simulink model "DatePersonalizate"  (R2023b)
settings: Solver=ode3  StartTime=0.0  StopTime=1000  FixedStep=0.1  RelTol=1e-3
values from neighbouring files (symbols this model uses):
  C = 7.4    [date_personalizate.m]
  k = 0.036    [date_personalizate.m]    (also in grafice.m = 0.035)
  k1 = 0.624    [date_personalizate.m]    (also in grafice.m)
  k11 = k2^2+4*(k-k3)*k1    (= 0.0915786)    [date_personalizate.m]
  k12 = 8*(k-k3)    (= 0.2928)    [date_personalizate.m]
  k13 = 2*(k-k3)    (= 0.0732)    [date_personalizate.m]
  k2 = -0.015    [date_personalizate.m]    (also in grafice.m)
  k3 = -0.0006    [date_personalizate.m]    (also in grafice.m)
  keta = 8e-5    (= 8e-05)    [date_personalizate.m]
  S = 332.5    [date_personalizate.m]
libraries: slpidlib x14, instrumentlib x2, simulink x1
(part 1 of 2)
settings Model: Creator=40787  LastModifiedBy=40787
settings GRTTargetCC: RTWCAPISignals=on  RTWCAPIParams=on

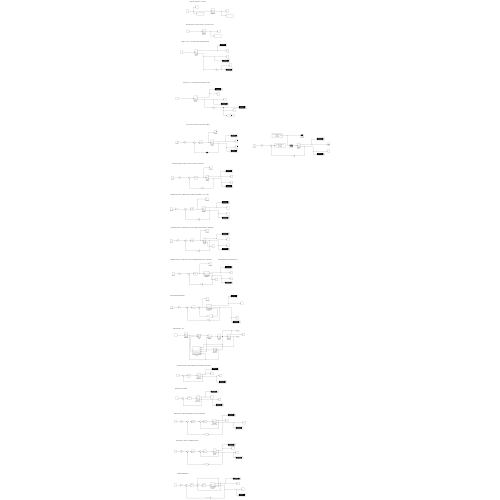
[thumbnail: Simulink's stored preview of the top-level diagram]
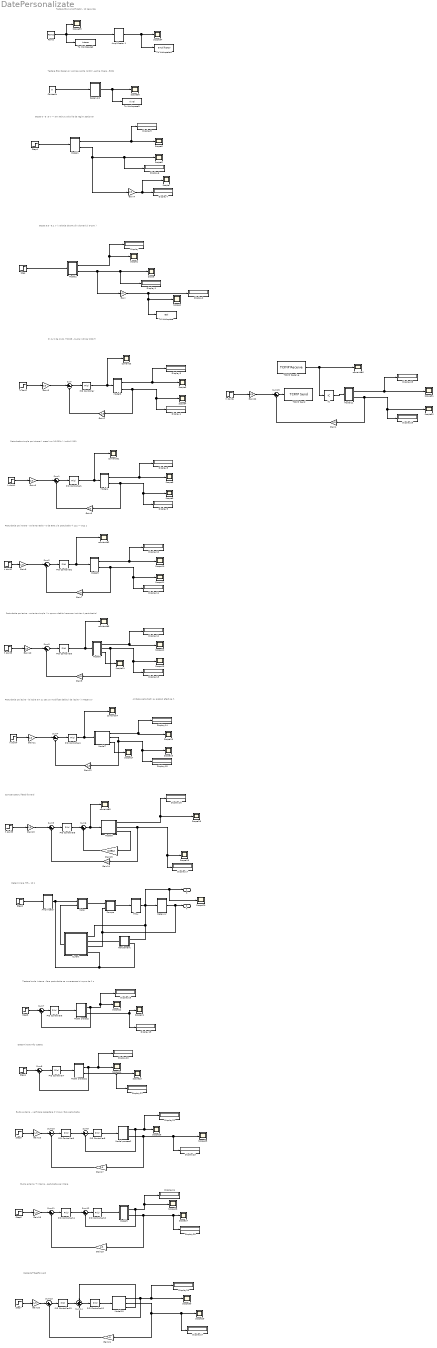
== system DatePersonalizate ==
  note: Testare Bloc Rezervor: pompa oprita (qi=0) - golire libera - 500s
  note: Testare Bloc Amplificator - 10 secunde
  note: trepta 0 - 5 .6 V -> am retinut valorile de regim stationar
  note: trepta 5.6 - 6.1 V ( variatie de 5% din domeniul 0-10V )
  note: PI cu tr de 112s, T0=28 - bucla inchisa (202/7)
  note: Perturbatie simpla pe intrare-> cresc k cu 10-20%-> inchid V101
  note: Perturbatie pe intrare - varianta reala - tr de 800 s la pertubatie + 112 -> 912 s
  note: Perturbatie pe iesire - varianta simpla ( in qe am debitul care era inainte + perturbatia)
  note: Perturbatie pe iesire - la iesire am cu cat s a modificat debitul de iesire - in Rezervor
  note: Compensatorul feed forward
  note: Determinare Hf1 - 10 s
  note: Testare bucla interna - fara perturbatie sa urmareasca tr impus de 1 s
  note: Determinare Hf2 -2500s
  note: Bucla externa - verificare respectare tr impus, fara perturbatie
  note: Bucla externa + interna - pertubatie pe intrare
  note: Cascada+feedforward
  note: Ambele perturbatii au acelasi efect pe h
  "Amplificator " : Subsystem
  Amplificator 1 : Subsystem
  Constant : Constant  Value=0
  Curent : Subsystem
  Display{,1..29} (30 alike) : Display
  Filtru : Subsystem
  Gain{,1..14,16..22} (22 alike) : Gain  Gain=1/3
  Gain15 : Gain  Gain=0.0912
  IC : InitialCondition  Value=5.6
  Model process : Subsystem
  Model process1 : Subsystem
  Model process2 : Subsystem
  Model1 : Subsystem
  Model10 : Subsystem
  Model11 : Subsystem
  Model2 : Subsystem
  Model3 : Subsystem
  Model4 : Subsystem
  Model5 : Subsystem
  Model6 : Subsystem
  Model7 : Subsystem
  Model8 : Subsystem
  Model9 : Subsystem
  Motor : Subsystem
  PID Controller{,1..5} (6 alike) : slpidlib/PID Controller  Controller=PI  Form=Parallel  TimeDomain=Continuous-time  UseExternalTs=off  SampleTime=-1  IntegratorMethod=Forward Euler  FilterMethod=Forward Euler  ControllerParametersSource=internal  P=2.96  I=2.96/202  UseKiTs=off  D=0  N=100  UseFilter=on  TunerSelectOption=Frequency Response Based  InitialConditionSource=internal  InitialConditionForIntegrator=5.6  InitialConditionForFilter=0  DifferentiatorICPrevScaledInput=0  ExternalReset=none  TrackingMode=off  Kt=1  LimitOutput=off  SatLimitsSource=internal  UpperSaturationLimit=inf  LowerSaturationLimit=-inf  LinearizeAsGain=on  AntiWindupMode=none  Kb=1  LimitIntegrator=off  UpperIntegratorSaturationLimit=inf  LowerIntegratorSaturationLimit=-inf  POutMin=[]  POutMax=[]  IOutMin=[]  IOutMax=[]  DOutMin=[]  DOutMax=[]  NOutMin=[]  NOutMax=[]  SumOutMin=[]  SumOutMax=[]  SaturationOutMin=[]  SaturationOutMax=[]  PParamMin=[]  PParamMax=[]  IParamMin=[]  IParamMax=[]  DParamMin=[]  DParamMax=[]  NParamMin=[]  NParamMax=[]  KbParamMin=[]  KbParamMax=[]  KtParamMin=[]  KtParamMax=[]  KbOutMin=[]  KbOutMax=[]  KtOutMin=[]  KtOutMax=[]  IntegratorOutMin=[]  IntegratorOutMax=[]  FilterOutMin=[]  FilterOutMax=[]  SumI1OutMin=[]  SumI1OutMax=[]  SumI2OutMin=[]  SumI2OutMax=[]  SumI3OutMin=[]  SumI3OutMax=[]  SumI4OutMin=[]  SumI4OutMax=[]  SumDOutMin=[]  SumDOutMax=[]  DifferentiatorOutMin=[]  DifferentiatorOutMax=[]  FilterDiffOutCoefMin=[]  FilterDiffOutCoefMax=[]  ReciprocalOutMin=[]  ReciprocalOutMax=[]  SumDenOutMin=[]  SumDenOutMax=[]  SumNumOutMin=[]  SumNumOutMax=[]  DivideOutMin=[]  DivideOutMax=[]  UdiffTsProdOutMin=[]  UdiffTsProdOutMax=[]  NTsProdOutMin=[]  NTsProdOutMax=[]  UintegralTsProdOutMin=[]  UintegralTsProdOutMax=[]  UngainTsProdOutMin=[]  UngainTsProdOutMax=[]  ClampingZeroOutDataTypeStr=Inherit: Inherit via back propagation  ClampingZeroOutMin=[]  ClampingZeroOutMax=[]  FilterDenConstantOutDataTypeStr=Inherit: Inherit via back propagation  FilterDenConstantOutMin=[]  FilterDenConstantOutMax=[]  PCopyOutDataTypeStr=Inherit: Inherit via back propagation  PCopyOutMin=[]  PCopyOutMax=[]  NCopyOutDataTypeStr=Inherit: Inherit via back propagation  NCopyOutMin=[]  NCopyOutMax=[]  IntegratorContinuousStateAttributes=''  IntegratorStateMustResolveToSignalObject=off  IntegratorRTWStateStorageClass=Auto  FilterContinuousStateAttributes=''  FilterStateMustResolveToSignalObject=off  FilterRTWStateStorageClass=Auto  ParallelPVariant=InternalParameters  IdealPVariant=Disabled  IVariant=InternalParameters  DVariant=Disabled  IntegratorVariant=Continuous  SatVariant=Disabled  AWVariant=Passthrough  PCopyVariant=Disabled  TRVariant=Disabled  FdbkBlocksVariant=Forward  IdealPFdbkVariant=Disabled  SatFdbkVariant=Disabled  DerivativeFilterVariant=Disabled  NVariant=Disabled  NCopyVariant=Disabled_SignalSpec  FilterICVariant=Disabled  IntegratorICVariant=InternalICs  ExternalResetVariant=Disabled  TRSumVariant=Passthrough  SumFdbkVariant=Disabled  SumVariant=Sum_PI  TsampFilterVariant=InternalTs  TsampNgainVariant=Passthrough  TsampIntegralVariant=Disabled_SignalSpec  ExternalSaturationOutDataTypeStr=Inherit: Same as second input
  PID Controller10 : slpidlib/PID Controller  Controller=PI  Form=Parallel  TimeDomain=Continuous-time  UseExternalTs=off  SampleTime=-1  IntegratorMethod=Forward Euler  FilterMethod=Forward Euler  ControllerParametersSource=internal  P=0.235  I=0.235/0.66  UseKiTs=off  D=0  N=100  UseFilter=on  TunerSelectOption=Frequency Response Based  InitialConditionSource=internal  InitialConditionForIntegrator=5.6  InitialConditionForFilter=0  DifferentiatorICPrevScaledInput=0  ExternalReset=none  TrackingMode=off  Kt=1  LimitOutput=off  SatLimitsSource=internal  UpperSaturationLimit=inf  LowerSaturationLimit=-inf  LinearizeAsGain=on  AntiWindupMode=none  Kb=1  LimitIntegrator=off  UpperIntegratorSaturationLimit=inf  LowerIntegratorSaturationLimit=-inf  POutMin=[]  POutMax=[]  IOutMin=[]  IOutMax=[]  DOutMin=[]  DOutMax=[]  NOutMin=[]  NOutMax=[]  SumOutMin=[]  SumOutMax=[]  SaturationOutMin=[]  SaturationOutMax=[]  PParamMin=[]  PParamMax=[]  IParamMin=[]  IParamMax=[]  DParamMin=[]  DParamMax=[]  NParamMin=[]  NParamMax=[]  KbParamMin=[]  KbParamMax=[]  KtParamMin=[]  KtParamMax=[]  KbOutMin=[]  KbOutMax=[]  KtOutMin=[]  KtOutMax=[]  IntegratorOutMin=[]  IntegratorOutMax=[]  FilterOutMin=[]  FilterOutMax=[]  SumI1OutMin=[]  SumI1OutMax=[]  SumI2OutMin=[]  SumI2OutMax=[]  SumI3OutMin=[]  SumI3OutMax=[]  SumI4OutMin=[]  SumI4OutMax=[]  SumDOutMin=[]  SumDOutMax=[]  DifferentiatorOutMin=[]  DifferentiatorOutMax=[]  FilterDiffOutCoefMin=[]  FilterDiffOutCoefMax=[]  ReciprocalOutMin=[]  ReciprocalOutMax=[]  SumDenOutMin=[]  SumDenOutMax=[]  SumNumOutMin=[]  SumNumOutMax=[]  DivideOutMin=[]  DivideOutMax=[]  UdiffTsProdOutMin=[]  UdiffTsProdOutMax=[]  NTsProdOutMin=[]  NTsProdOutMax=[]  UintegralTsProdOutMin=[]  UintegralTsProdOutMax=[]  UngainTsProdOutMin=[]  UngainTsProdOutMax=[]  ClampingZeroOutDataTypeStr=Inherit: Inherit via back propagation  ClampingZeroOutMin=[]  ClampingZeroOutMax=[]  FilterDenConstantOutDataTypeStr=Inherit: Inherit via back propagation  FilterDenConstantOutMin=[]  FilterDenConstantOutMax=[]  PCopyOutDataTypeStr=Inherit: Inherit via back propagation  PCopyOutMin=[]  PCopyOutMax=[]  NCopyOutDataTypeStr=Inherit: Inherit via back propagation  NCopyOutMin=[]  NCopyOutMax=[]  IntegratorContinuousStateAttributes=''  IntegratorStateMustResolveToSignalObject=off  IntegratorRTWStateStorageClass=Auto  FilterContinuousStateAttributes=''  FilterStateMustResolveToSignalObject=off  FilterRTWStateStorageClass=Auto  ParallelPVariant=InternalParameters  IdealPVariant=Disabled  IVariant=InternalParameters  DVariant=Disabled  IntegratorVariant=Continuous  SatVariant=Disabled  AWVariant=Passthrough  PCopyVariant=Disabled  TRVariant=Disabled  FdbkBlocksVariant=Forward  IdealPFdbkVariant=Disabled  SatFdbkVariant=Disabled  DerivativeFilterVariant=Disabled  NVariant=Disabled  NCopyVariant=Disabled_SignalSpec  FilterICVariant=Disabled  IntegratorICVariant=InternalICs  ExternalResetVariant=Disabled  TRSumVariant=Passthrough  SumFdbkVariant=Disabled  SumVariant=Sum_PI  TsampFilterVariant=InternalTs  TsampNgainVariant=Passthrough  TsampIntegralVariant=Disabled_SignalSpec  ExternalSaturationOutDataTypeStr=Inherit: Same as second input
  PID Controller11 : slpidlib/PID Controller  Controller=PI  Form=Parallel  TimeDomain=Continuous-time  UseExternalTs=off  SampleTime=-1  IntegratorMethod=Forward Euler  FilterMethod=Forward Euler  ControllerParametersSource=internal  P=39  I=39/404  UseKiTs=off  D=0  N=100  UseFilter=on  TunerSelectOption=Frequency Response Based  InitialConditionSource=internal  InitialConditionForIntegrator=30.22  InitialConditionForFilter=0  DifferentiatorICPrevScaledInput=0  ExternalReset=none  TrackingMode=off  Kt=1  LimitOutput=off  SatLimitsSource=internal  UpperSaturationLimit=inf  LowerSaturationLimit=-inf  LinearizeAsGain=on  AntiWindupMode=none  Kb=1  LimitIntegrator=off  UpperIntegratorSaturationLimit=inf  LowerIntegratorSaturationLimit=-inf  POutMin=[]  POutMax=[]  IOutMin=[]  IOutMax=[]  DOutMin=[]  DOutMax=[]  NOutMin=[]  NOutMax=[]  SumOutMin=[]  SumOutMax=[]  SaturationOutMin=[]  SaturationOutMax=[]  PParamMin=[]  PParamMax=[]  IParamMin=[]  IParamMax=[]  DParamMin=[]  DParamMax=[]  NParamMin=[]  NParamMax=[]  KbParamMin=[]  KbParamMax=[]  KtParamMin=[]  KtParamMax=[]  KbOutMin=[]  KbOutMax=[]  KtOutMin=[]  KtOutMax=[]  IntegratorOutMin=[]  IntegratorOutMax=[]  FilterOutMin=[]  FilterOutMax=[]  SumI1OutMin=[]  SumI1OutMax=[]  SumI2OutMin=[]  SumI2OutMax=[]  SumI3OutMin=[]  SumI3OutMax=[]  SumI4OutMin=[]  SumI4OutMax=[]  SumDOutMin=[]  SumDOutMax=[]  DifferentiatorOutMin=[]  DifferentiatorOutMax=[]  FilterDiffOutCoefMin=[]  FilterDiffOutCoefMax=[]  ReciprocalOutMin=[]  ReciprocalOutMax=[]  SumDenOutMin=[]  SumDenOutMax=[]  SumNumOutMin=[]  SumNumOutMax=[]  DivideOutMin=[]  DivideOutMax=[]  UdiffTsProdOutMin=[]  UdiffTsProdOutMax=[]  NTsProdOutMin=[]  NTsProdOutMax=[]  UintegralTsProdOutMin=[]  UintegralTsProdOutMax=[]  UngainTsProdOutMin=[]  UngainTsProdOutMax=[]  ClampingZeroOutDataTypeStr=Inherit: Inherit via back propagation  ClampingZeroOutMin=[]  ClampingZeroOutMax=[]  FilterDenConstantOutDataTypeStr=Inherit: Inherit via back propagation  FilterDenConstantOutMin=[]  FilterDenConstantOutMax=[]  PCopyOutDataTypeStr=Inherit: Inherit via back propagation  PCopyOutMin=[]  PCopyOutMax=[]  NCopyOutDataTypeStr=Inherit: Inherit via back propagation  NCopyOutMin=[]  NCopyOutMax=[]  IntegratorContinuousStateAttributes=''  IntegratorStateMustResolveToSignalObject=off  IntegratorRTWStateStorageClass=Auto  FilterContinuousStateAttributes=''  FilterStateMustResolveToSignalObject=off  FilterRTWStateStorageClass=Auto  ParallelPVariant=InternalParameters  IdealPVariant=Disabled  IVariant=InternalParameters  DVariant=Disabled  IntegratorVariant=Continuous  SatVariant=Disabled  AWVariant=Passthrough  PCopyVariant=Disabled  TRVariant=Disabled  FdbkBlocksVariant=Forward  IdealPFdbkVariant=Disabled  SatFdbkVariant=Disabled  DerivativeFilterVariant=Disabled  NVariant=Disabled  NCopyVariant=Disabled_SignalSpec  FilterICVariant=Disabled  IntegratorICVariant=InternalICs  ExternalResetVariant=Disabled  TRSumVariant=Passthrough  SumFdbkVariant=Disabled  SumVariant=Sum_PI  TsampFilterVariant=InternalTs  TsampNgainVariant=Passthrough  TsampIntegralVariant=Disabled_SignalSpec  ExternalSaturationOutDataTypeStr=Inherit: Same as second input
  PID Controller12 : slpidlib/PID Controller  Controller=PI  Form=Parallel  TimeDomain=Continuous-time  UseExternalTs=off  SampleTime=-1  IntegratorMethod=Forward Euler  FilterMethod=Forward Euler  ControllerParametersSource=internal  P=0.235  I=0.235/0.66  UseKiTs=off  D=0  N=100  UseFilter=on  TunerSelectOption=Frequency Response Based  InitialConditionSource=internal  InitialConditionForIntegrator=5.6  InitialConditionForFilter=0  DifferentiatorICPrevScaledInput=0  ExternalReset=none  TrackingMode=off  Kt=1  LimitOutput=off  SatLimitsSource=internal  UpperSaturationLimit=inf  LowerSaturationLimit=-inf  LinearizeAsGain=on  AntiWindupMode=none  Kb=1  LimitIntegrator=off  UpperIntegratorSaturationLimit=inf  LowerIntegratorSaturationLimit=-inf  POutMin=[]  POutMax=[]  IOutMin=[]  IOutMax=[]  DOutMin=[]  DOutMax=[]  NOutMin=[]  NOutMax=[]  SumOutMin=[]  SumOutMax=[]  SaturationOutMin=[]  SaturationOutMax=[]  PParamMin=[]  PParamMax=[]  IParamMin=[]  IParamMax=[]  DParamMin=[]  DParamMax=[]  NParamMin=[]  NParamMax=[]  KbParamMin=[]  KbParamMax=[]  KtParamMin=[]  KtParamMax=[]  KbOutMin=[]  KbOutMax=[]  KtOutMin=[]  KtOutMax=[]  IntegratorOutMin=[]  IntegratorOutMax=[]  FilterOutMin=[]  FilterOutMax=[]  SumI1OutMin=[]  SumI1OutMax=[]  SumI2OutMin=[]  SumI2OutMax=[]  SumI3OutMin=[]  SumI3OutMax=[]  SumI4OutMin=[]  SumI4OutMax=[]  SumDOutMin=[]  SumDOutMax=[]  DifferentiatorOutMin=[]  DifferentiatorOutMax=[]  FilterDiffOutCoefMin=[]  FilterDiffOutCoefMax=[]  ReciprocalOutMin=[]  ReciprocalOutMax=[]  SumDenOutMin=[]  SumDenOutMax=[]  SumNumOutMin=[]  SumNumOutMax=[]  DivideOutMin=[]  DivideOutMax=[]  UdiffTsProdOutMin=[]  UdiffTsProdOutMax=[]  NTsProdOutMin=[]  NTsProdOutMax=[]  UintegralTsProdOutMin=[]  UintegralTsProdOutMax=[]  UngainTsProdOutMin=[]  UngainTsProdOutMax=[]  ClampingZeroOutDataTypeStr=Inherit: Inherit via back propagation  ClampingZeroOutMin=[]  ClampingZeroOutMax=[]  FilterDenConstantOutDataTypeStr=Inherit: Inherit via back propagation  FilterDenConstantOutMin=[]  FilterDenConstantOutMax=[]  PCopyOutDataTypeStr=Inherit: Inherit via back propagation  PCopyOutMin=[]  PCopyOutMax=[]  NCopyOutDataTypeStr=Inherit: Inherit via back propagation  NCopyOutMin=[]  NCopyOutMax=[]  IntegratorContinuousStateAttributes=''  IntegratorStateMustResolveToSignalObject=off  IntegratorRTWStateStorageClass=Auto  FilterContinuousStateAttributes=''  FilterStateMustResolveToSignalObject=off  FilterRTWStateStorageClass=Auto  ParallelPVariant=InternalParameters  IdealPVariant=Disabled  IVariant=InternalParameters  DVariant=Disabled  IntegratorVariant=Continuous  SatVariant=Disabled  AWVariant=Passthrough  PCopyVariant=Disabled  TRVariant=Disabled  FdbkBlocksVariant=Forward  IdealPFdbkVariant=Disabled  SatFdbkVariant=Disabled  DerivativeFilterVariant=Disabled  NVariant=Disabled  NCopyVariant=Disabled_SignalSpec  FilterICVariant=Disabled  IntegratorICVariant=InternalICs  ExternalResetVariant=Disabled  TRSumVariant=Passthrough  SumFdbkVariant=Disabled  SumVariant=Sum_PI  TsampFilterVariant=InternalTs  TsampNgainVariant=Passthrough  TsampIntegralVariant=Disabled_SignalSpec  ExternalSaturationOutDataTypeStr=Inherit: Same as second input
  PID Controller13 : slpidlib/PID Controller  Controller=PI  Form=Parallel  TimeDomain=Continuous-time  UseExternalTs=off  SampleTime=-1  IntegratorMethod=Forward Euler  FilterMethod=Forward Euler  ControllerParametersSource=internal  P=6.58  I=6.58/404  UseKiTs=off  D=0  N=100  UseFilter=on  TunerSelectOption=Frequency Response Based  InitialConditionSource=internal  InitialConditionForIntegrator=30.22  InitialConditionForFilter=0  DifferentiatorICPrevScaledInput=0  ExternalReset=none  TrackingMode=off  Kt=1  LimitOutput=off  SatLimitsSource=internal  UpperSaturationLimit=inf  LowerSaturationLimit=-inf  LinearizeAsGain=on  AntiWindupMode=none  Kb=1  LimitIntegrator=off  UpperIntegratorSaturationLimit=inf  LowerIntegratorSaturationLimit=-inf  POutMin=[]  POutMax=[]  IOutMin=[]  IOutMax=[]  DOutMin=[]  DOutMax=[]  NOutMin=[]  NOutMax=[]  SumOutMin=[]  SumOutMax=[]  SaturationOutMin=[]  SaturationOutMax=[]  PParamMin=[]  PParamMax=[]  IParamMin=[]  IParamMax=[]  DParamMin=[]  DParamMax=[]  NParamMin=[]  NParamMax=[]  KbParamMin=[]  KbParamMax=[]  KtParamMin=[]  KtParamMax=[]  KbOutMin=[]  KbOutMax=[]  KtOutMin=[]  KtOutMax=[]  IntegratorOutMin=[]  IntegratorOutMax=[]  FilterOutMin=[]  FilterOutMax=[]  SumI1OutMin=[]  SumI1OutMax=[]  SumI2OutMin=[]  SumI2OutMax=[]  SumI3OutMin=[]  SumI3OutMax=[]  SumI4OutMin=[]  SumI4OutMax=[]  SumDOutMin=[]  SumDOutMax=[]  DifferentiatorOutMin=[]  DifferentiatorOutMax=[]  FilterDiffOutCoefMin=[]  FilterDiffOutCoefMax=[]  ReciprocalOutMin=[]  ReciprocalOutMax=[]  SumDenOutMin=[]  SumDenOutMax=[]  SumNumOutMin=[]  SumNumOutMax=[]  DivideOutMin=[]  DivideOutMax=[]  UdiffTsProdOutMin=[]  UdiffTsProdOutMax=[]  NTsProdOutMin=[]  NTsProdOutMax=[]  UintegralTsProdOutMin=[]  UintegralTsProdOutMax=[]  UngainTsProdOutMin=[]  UngainTsProdOutMax=[]  ClampingZeroOutDataTypeStr=Inherit: Inherit via back propagation  ClampingZeroOutMin=[]  ClampingZeroOutMax=[]  FilterDenConstantOutDataTypeStr=Inherit: Inherit via back propagation  FilterDenConstantOutMin=[]  FilterDenConstantOutMax=[]  PCopyOutDataTypeStr=Inherit: Inherit via back propagation  PCopyOutMin=[]  PCopyOutMax=[]  NCopyOutDataTypeStr=Inherit: Inherit via back propagation  NCopyOutMin=[]  NCopyOutMax=[]  IntegratorContinuousStateAttributes=''  IntegratorStateMustResolveToSignalObject=off  IntegratorRTWStateStorageClass=Auto  FilterContinuousStateAttributes=''  FilterStateMustResolveToSignalObject=off  FilterRTWStateStorageClass=Auto  ParallelPVariant=InternalParameters  IdealPVariant=Disabled  IVariant=InternalParameters  DVariant=Disabled  IntegratorVariant=Continuous  SatVariant=Disabled  AWVariant=Passthrough  PCopyVariant=Disabled  TRVariant=Disabled  FdbkBlocksVariant=Forward  IdealPFdbkVariant=Disabled  SatFdbkVariant=Disabled  DerivativeFilterVariant=Disabled  NVariant=Disabled  NCopyVariant=Disabled_SignalSpec  FilterICVariant=Disabled  IntegratorICVariant=InternalICs  ExternalResetVariant=Disabled  TRSumVariant=Passthrough  SumFdbkVariant=Disabled  SumVariant=Sum_PI  TsampFilterVariant=InternalTs  TsampNgainVariant=Passthrough  TsampIntegralVariant=Disabled_SignalSpec  ExternalSaturationOutDataTypeStr=Inherit: Same as second input
  PID Controller6 : slpidlib/PID Controller  Controller=PI  Form=Parallel  TimeDomain=Continuous-time  UseExternalTs=off  SampleTime=-1  IntegratorMethod=Forward Euler  FilterMethod=Forward Euler  ControllerParametersSource=internal  P=0.277  I=0.277/0.76  UseKiTs=off  D=0  N=100  UseFilter=on  TunerSelectOption=Frequency Response Based  InitialConditionSource=internal  InitialConditionForIntegrator=5.6  InitialConditionForFilter=0  DifferentiatorICPrevScaledInput=0  ExternalReset=none  TrackingMode=off  Kt=1  LimitOutput=off  SatLimitsSource=internal  UpperSaturationLimit=inf  LowerSaturationLimit=-inf  LinearizeAsGain=on  AntiWindupMode=none  Kb=1  LimitIntegrator=off  UpperIntegratorSaturationLimit=inf  LowerIntegratorSaturationLimit=-inf  POutMin=[]  POutMax=[]  IOutMin=[]  IOutMax=[]  DOutMin=[]  DOutMax=[]  NOutMin=[]  NOutMax=[]  SumOutMin=[]  SumOutMax=[]  SaturationOutMin=[]  SaturationOutMax=[]  PParamMin=[]  PParamMax=[]  IParamMin=[]  IParamMax=[]  DParamMin=[]  DParamMax=[]  NParamMin=[]  NParamMax=[]  KbParamMin=[]  KbParamMax=[]  KtParamMin=[]  KtParamMax=[]  KbOutMin=[]  KbOutMax=[]  KtOutMin=[]  KtOutMax=[]  IntegratorOutMin=[]  IntegratorOutMax=[]  FilterOutMin=[]  FilterOutMax=[]  SumI1OutMin=[]  SumI1OutMax=[]  SumI2OutMin=[]  SumI2OutMax=[]  SumI3OutMin=[]  SumI3OutMax=[]  SumI4OutMin=[]  SumI4OutMax=[]  SumDOutMin=[]  SumDOutMax=[]  DifferentiatorOutMin=[]  DifferentiatorOutMax=[]  FilterDiffOutCoefMin=[]  FilterDiffOutCoefMax=[]  ReciprocalOutMin=[]  ReciprocalOutMax=[]  SumDenOutMin=[]  SumDenOutMax=[]  SumNumOutMin=[]  SumNumOutMax=[]  DivideOutMin=[]  DivideOutMax=[]  UdiffTsProdOutMin=[]  UdiffTsProdOutMax=[]  NTsProdOutMin=[]  NTsProdOutMax=[]  UintegralTsProdOutMin=[]  UintegralTsProdOutMax=[]  UngainTsProdOutMin=[]  UngainTsProdOutMax=[]  ClampingZeroOutDataTypeStr=Inherit: Inherit via back propagation  ClampingZeroOutMin=[]  ClampingZeroOutMax=[]  FilterDenConstantOutDataTypeStr=Inherit: Inherit via back propagation  FilterDenConstantOutMin=[]  FilterDenConstantOutMax=[]  PCopyOutDataTypeStr=Inherit: Inherit via back propagation  PCopyOutMin=[]  PCopyOutMax=[]  NCopyOutDataTypeStr=Inherit: Inherit via back propagation  NCopyOutMin=[]  NCopyOutMax=[]  IntegratorContinuousStateAttributes=''  IntegratorStateMustResolveToSignalObject=off  IntegratorRTWStateStorageClass=Auto  FilterContinuousStateAttributes=''  FilterStateMustResolveToSignalObject=off  FilterRTWStateStorageClass=Auto  ParallelPVariant=InternalParameters  IdealPVariant=Disabled  IVariant=InternalParameters  DVariant=Disabled  IntegratorVariant=Continuous  SatVariant=Disabled  AWVariant=Passthrough  PCopyVariant=Disabled  TRVariant=Disabled  FdbkBlocksVariant=Forward  IdealPFdbkVariant=Disabled  SatFdbkVariant=Disabled  DerivativeFilterVariant=Disabled  NVariant=Disabled  NCopyVariant=Disabled_SignalSpec  FilterICVariant=Disabled  IntegratorICVariant=InternalICs  ExternalResetVariant=Disabled  TRSumVariant=Passthrough  SumFdbkVariant=Disabled  SumVariant=Sum_PI  TsampFilterVariant=InternalTs  TsampNgainVariant=Passthrough  TsampIntegralVariant=Disabled_SignalSpec  ExternalSaturationOutDataTypeStr=Inherit: Same as second input
  PID Controller7 : slpidlib/PID Controller  Controller=PI  Form=Parallel  TimeDomain=Continuous-time  UseExternalTs=off  SampleTime=-1  IntegratorMethod=Forward Euler  FilterMethod=Forward Euler  ControllerParametersSource=internal  P=0.277  I=0.277/0.76  UseKiTs=off  D=0  N=100  UseFilter=on  TunerSelectOption=Frequency Response Based  InitialConditionSource=internal  InitialConditionForIntegrator=5.6  InitialConditionForFilter=0  DifferentiatorICPrevScaledInput=0  ExternalReset=none  TrackingMode=off  Kt=1  LimitOutput=off  SatLimitsSource=internal  UpperSaturationLimit=inf  LowerSaturationLimit=-inf  LinearizeAsGain=on  AntiWindupMode=none  Kb=1  LimitIntegrator=off  UpperIntegratorSaturationLimit=inf  LowerIntegratorSaturationLimit=-inf  POutMin=[]  POutMax=[]  IOutMin=[]  IOutMax=[]  DOutMin=[]  DOutMax=[]  NOutMin=[]  NOutMax=[]  SumOutMin=[]  SumOutMax=[]  SaturationOutMin=[]  SaturationOutMax=[]  PParamMin=[]  PParamMax=[]  IParamMin=[]  IParamMax=[]  DParamMin=[]  DParamMax=[]  NParamMin=[]  NParamMax=[]  KbParamMin=[]  KbParamMax=[]  KtParamMin=[]  KtParamMax=[]  KbOutMin=[]  KbOutMax=[]  KtOutMin=[]  KtOutMax=[]  IntegratorOutMin=[]  IntegratorOutMax=[]  FilterOutMin=[]  FilterOutMax=[]  SumI1OutMin=[]  SumI1OutMax=[]  SumI2OutMin=[]  SumI2OutMax=[]  SumI3OutMin=[]  SumI3OutMax=[]  SumI4OutMin=[]  SumI4OutMax=[]  SumDOutMin=[]  SumDOutMax=[]  DifferentiatorOutMin=[]  DifferentiatorOutMax=[]  FilterDiffOutCoefMin=[]  FilterDiffOutCoefMax=[]  ReciprocalOutMin=[]  ReciprocalOutMax=[]  SumDenOutMin=[]  SumDenOutMax=[]  SumNumOutMin=[]  SumNumOutMax=[]  DivideOutMin=[]  DivideOutMax=[]  UdiffTsProdOutMin=[]  UdiffTsProdOutMax=[]  NTsProdOutMin=[]  NTsProdOutMax=[]  UintegralTsProdOutMin=[]  UintegralTsProdOutMax=[]  UngainTsProdOutMin=[]  UngainTsProdOutMax=[]  ClampingZeroOutDataTypeStr=Inherit: Inherit via back propagation  ClampingZeroOutMin=[]  ClampingZeroOutMax=[]  FilterDenConstantOutDataTypeStr=Inherit: Inherit via back propagation  FilterDenConstantOutMin=[]  FilterDenConstantOutMax=[]  PCopyOutDataTypeStr=Inherit: Inherit via back propagation  PCopyOutMin=[]  PCopyOutMax=[]  NCopyOutDataTypeStr=Inherit: Inherit via back propagation  NCopyOutMin=[]  NCopyOutMax=[]  IntegratorContinuousStateAttributes=''  IntegratorStateMustResolveToSignalObject=off  IntegratorRTWStateStorageClass=Auto  FilterContinuousStateAttributes=''  FilterStateMustResolveToSignalObject=off  FilterRTWStateStorageClass=Auto  ParallelPVariant=InternalParameters  IdealPVariant=Disabled  IVariant=InternalParameters  DVariant=Disabled  IntegratorVariant=Continuous  SatVariant=Disabled  AWVariant=Passthrough  PCopyVariant=Disabled  TRVariant=Disabled  FdbkBlocksVariant=Forward  IdealPFdbkVariant=Disabled  SatFdbkVariant=Disabled  DerivativeFilterVariant=Disabled  NVariant=Disabled  NCopyVariant=Disabled_SignalSpec  FilterICVariant=Disabled  IntegratorICVariant=InternalICs  ExternalResetVariant=Disabled  TRSumVariant=Passthrough  SumFdbkVariant=Disabled  SumVariant=Sum_PI  TsampFilterVariant=InternalTs  TsampNgainVariant=Passthrough  TsampIntegralVariant=Disabled_SignalSpec  ExternalSaturationOutDataTypeStr=Inherit: Same as second input
  PID Controller8 : slpidlib/PID Controller  Controller=PI  Form=Parallel  TimeDomain=Continuous-time  UseExternalTs=off  SampleTime=-1  IntegratorMethod=Forward Euler  FilterMethod=Forward Euler  ControllerParametersSource=internal  P=0.235  I=0.235/0.66  UseKiTs=off  D=0  N=100  UseFilter=on  TunerSelectOption=Frequency Response Based  InitialConditionSource=internal  InitialConditionForIntegrator=5.6  InitialConditionForFilter=0  DifferentiatorICPrevScaledInput=0  ExternalReset=none  TrackingMode=off  Kt=1  LimitOutput=off  SatLimitsSource=internal  UpperSaturationLimit=inf  LowerSaturationLimit=-inf  LinearizeAsGain=on  AntiWindupMode=none  Kb=1  LimitIntegrator=off  UpperIntegratorSaturationLimit=inf  LowerIntegratorSaturationLimit=-inf  POutMin=[]  POutMax=[]  IOutMin=[]  IOutMax=[]  DOutMin=[]  DOutMax=[]  NOutMin=[]  NOutMax=[]  SumOutMin=[]  SumOutMax=[]  SaturationOutMin=[]  SaturationOutMax=[]  PParamMin=[]  PParamMax=[]  IParamMin=[]  IParamMax=[]  DParamMin=[]  DParamMax=[]  NParamMin=[]  NParamMax=[]  KbParamMin=[]  KbParamMax=[]  KtParamMin=[]  KtParamMax=[]  KbOutMin=[]  KbOutMax=[]  KtOutMin=[]  KtOutMax=[]  IntegratorOutMin=[]  IntegratorOutMax=[]  FilterOutMin=[]  FilterOutMax=[]  SumI1OutMin=[]  SumI1OutMax=[]  SumI2OutMin=[]  SumI2OutMax=[]  SumI3OutMin=[]  SumI3OutMax=[]  SumI4OutMin=[]  SumI4OutMax=[]  SumDOutMin=[]  SumDOutMax=[]  DifferentiatorOutMin=[]  DifferentiatorOutMax=[]  FilterDiffOutCoefMin=[]  FilterDiffOutCoefMax=[]  ReciprocalOutMin=[]  ReciprocalOutMax=[]  SumDenOutMin=[]  SumDenOutMax=[]  SumNumOutMin=[]  SumNumOutMax=[]  DivideOutMin=[]  DivideOutMax=[]  UdiffTsProdOutMin=[]  UdiffTsProdOutMax=[]  NTsProdOutMin=[]  NTsProdOutMax=[]  UintegralTsProdOutMin=[]  UintegralTsProdOutMax=[]  UngainTsProdOutMin=[]  UngainTsProdOutMax=[]  ClampingZeroOutDataTypeStr=Inherit: Inherit via back propagation  ClampingZeroOutMin=[]  ClampingZeroOutMax=[]  FilterDenConstantOutDataTypeStr=Inherit: Inherit via back propagation  FilterDenConstantOutMin=[]  FilterDenConstantOutMax=[]  PCopyOutDataTypeStr=Inherit: Inherit via back propagation  PCopyOutMin=[]  PCopyOutMax=[]  NCopyOutDataTypeStr=Inherit: Inherit via back propagation  NCopyOutMin=[]  NCopyOutMax=[]  IntegratorContinuousStateAttributes=''  IntegratorStateMustResolveToSignalObject=off  IntegratorRTWStateStorageClass=Auto  FilterContinuousStateAttributes=''  FilterStateMustResolveToSignalObject=off  FilterRTWStateStorageClass=Auto  ParallelPVariant=InternalParameters  IdealPVariant=Disabled  IVariant=InternalParameters  DVariant=Disabled  IntegratorVariant=Continuous  SatVariant=Disabled  AWVariant=Passthrough  PCopyVariant=Disabled  TRVariant=Disabled  FdbkBlocksVariant=Forward  IdealPFdbkVariant=Disabled  SatFdbkVariant=Disabled  DerivativeFilterVariant=Disabled  NVariant=Disabled  NCopyVariant=Disabled_SignalSpec  FilterICVariant=Disabled  IntegratorICVariant=InternalICs  ExternalResetVariant=Disabled  TRSumVariant=Passthrough  SumFdbkVariant=Disabled  SumVariant=Sum_PI  TsampFilterVariant=InternalTs  TsampNgainVariant=Passthrough  TsampIntegralVariant=Disabled_SignalSpec  ExternalSaturationOutDataTypeStr=Inherit: Same as second input
  PID Controller9 : slpidlib/PID Controller  Controller=PI  Form=Parallel  TimeDomain=Continuous-time  UseExternalTs=off  SampleTime=-1  IntegratorMethod=Forward Euler  FilterMethod=Forward Euler  ControllerParametersSource=internal  P=39  I=39/404  UseKiTs=off  D=0  N=100  UseFilter=on  TunerSelectOption=Frequency Response Based  InitialConditionSource=internal  InitialConditionForIntegrator=30.22  InitialConditionForFilter=0  DifferentiatorICPrevScaledInput=0  ExternalReset=none  TrackingMode=off  Kt=1  LimitOutput=off  SatLimitsSource=internal  UpperSaturationLimit=inf  LowerSaturationLimit=-inf  LinearizeAsGain=on  AntiWindupMode=none  Kb=1  LimitIntegrator=off  UpperIntegratorSaturationLimit=inf  LowerIntegratorSaturationLimit=-inf  POutMin=[]  POutMax=[]  IOutMin=[]  IOutMax=[]  DOutMin=[]  DOutMax=[]  NOutMin=[]  NOutMax=[]  SumOutMin=[]  SumOutMax=[]  SaturationOutMin=[]  SaturationOutMax=[]  PParamMin=[]  PParamMax=[]  IParamMin=[]  IParamMax=[]  DParamMin=[]  DParamMax=[]  NParamMin=[]  NParamMax=[]  KbParamMin=[]  KbParamMax=[]  KtParamMin=[]  KtParamMax=[]  KbOutMin=[]  KbOutMax=[]  KtOutMin=[]  KtOutMax=[]  IntegratorOutMin=[]  IntegratorOutMax=[]  FilterOutMin=[]  FilterOutMax=[]  SumI1OutMin=[]  SumI1OutMax=[]  SumI2OutMin=[]  SumI2OutMax=[]  SumI3OutMin=[]  SumI3OutMax=[]  SumI4OutMin=[]  SumI4OutMax=[]  SumDOutMin=[]  SumDOutMax=[]  DifferentiatorOutMin=[]  DifferentiatorOutMax=[]  FilterDiffOutCoefMin=[]  FilterDiffOutCoefMax=[]  ReciprocalOutMin=[]  ReciprocalOutMax=[]  SumDenOutMin=[]  SumDenOutMax=[]  SumNumOutMin=[]  SumNumOutMax=[]  DivideOutMin=[]  DivideOutMax=[]  UdiffTsProdOutMin=[]  UdiffTsProdOutMax=[]  NTsProdOutMin=[]  NTsProdOutMax=[]  UintegralTsProdOutMin=[]  UintegralTsProdOutMax=[]  UngainTsProdOutMin=[]  UngainTsProdOutMax=[]  ClampingZeroOutDataTypeStr=Inherit: Inherit via back propagation  ClampingZeroOutMin=[]  ClampingZeroOutMax=[]  FilterDenConstantOutDataTypeStr=Inherit: Inherit via back propagation  FilterDenConstantOutMin=[]  FilterDenConstantOutMax=[]  PCopyOutDataTypeStr=Inherit: Inherit via back propagation  PCopyOutMin=[]  PCopyOutMax=[]  NCopyOutDataTypeStr=Inherit: Inherit via back propagation  NCopyOutMin=[]  NCopyOutMax=[]  IntegratorContinuousStateAttributes=''  IntegratorStateMustResolveToSignalObject=off  IntegratorRTWStateStorageClass=Auto  FilterContinuousStateAttributes=''  FilterStateMustResolveToSignalObject=off  FilterRTWStateStorageClass=Auto  ParallelPVariant=InternalParameters  IdealPVariant=Disabled  IVariant=InternalParameters  DVariant=Disabled  IntegratorVariant=Continuous  SatVariant=Disabled  AWVariant=Passthrough  PCopyVariant=Disabled  TRVariant=Disabled  FdbkBlocksVariant=Forward  IdealPFdbkVariant=Disabled  SatFdbkVariant=Disabled  DerivativeFilterVariant=Disabled  NVariant=Disabled  NCopyVariant=Disabled_SignalSpec  FilterICVariant=Disabled  IntegratorICVariant=InternalICs  ExternalResetVariant=Disabled  TRSumVariant=Passthrough  SumFdbkVariant=Disabled  SumVariant=Sum_PI  TsampFilterVariant=InternalTs  TsampNgainVariant=Passthrough  TsampIntegralVariant=Disabled_SignalSpec  ExternalSaturationOutDataTypeStr=Inherit: Same as second input
  Pompa : Subsystem
  Ramp : simulink/Sources/Ramp  slope=1  start=0  InitialOutput=0
  Randament : Subsystem
  Rezervor : Subsystem
  Rezervor1 : Subsystem
  Scope{,1..32,34..36} (36 alike) : Scope
  Step : Step  Time=0  Before=5.6  After=6.1  SampleTime=0
  Step1 : Step  Time=0  After=5.6  SampleTime=0
  Step2 : Step  Time=0  Before=5.6  After=6.1  SampleTime=0
  Step3 : Step  Time=0  Before=30.22  After=35.7  SampleTime=0
  Step4 : Step  Time=0  Before=30.22  After=35.7  SampleTime=0
  Step5 : Step  Time=0  After=20  SampleTime=0
  Step6 : Step  Time=0  After=20  SampleTime=0
  Step7 : Step  Time=0  After=20  SampleTime=0
  Sum{,1..5,7..13,15} (14 alike) : Sum  Inputs=|+-
  Sum14 : Sum  Inputs=++-
  Sum6 : Sum  Inputs=|++
  TCP/IP Receive : instrumentlib/TCP//IP Receive  Host=127.0.0.1  Port=5000  DataSize=1  DataType=double  ASCIIFormatting=%f  Terminator=LF  CustomTerminator=10  ByteOrder=little-endian  EnableBlockingMode=on  Timeout=10  SampleTime=0.1  SimulateUsing=Interpreted execution
  TCP/IP Send : instrumentlib/TCP//IP Send  Host=127.0.0.1  Port=5000  ByteOrder=little-endian  EnableBlockingMode=on  Timeout=10  TransferDelay=off  SimulateUsing=Interpreted execution
  To Workspace : ToWorkspace  VariableName=real  SampleTime=-1
  To Workspace1 : ToWorkspace  VariableName=amplificator  SampleTime=-1
  To Workspace2 : ToWorkspace  VariableName=intrare  SampleTime=-1
  To Workspace3 : ToWorkspace  VariableName=nivel  SampleTime=-1
  comanda{,1..6} (7 alike) : Scope
  h dorit{,1..6} (7 alike) : Step  Time=0  After=20  SampleTime=0
  q : Outport
  h : Outport  Port=2
  wires:
  Model2/2(h) -> Gain/1, Display1/1, Scope/1
  Model2/1(q) -> Display/1, Scope1/1
  Gain/1 -> To Workspace/1, Scope2/1, Display2/1
  Step/1 -> Model2/1(ua)
  Gain2/1 -> Sum/2
  h dorit/1 -> Gain3/1
  Sum/1 -> PID Controller/1
  Gain3/1 -> Sum/1
  PID Controller/1 -> Model3/1(ua), comanda/1
  Model3/2(h) -> Gain2/1, Display4/1, Scope4/1
  Model3/1(q) -> Scope3/1, Display3/1
  Gain4/1 -> Scope7/1, Display7/1
  Step1/1 -> Model1/1(ua)
  Model1/1(q) -> Display5/1, Scope6/1
  Model1/2(h) -> Gain4/1, Display6/1, Scope5/1
  Model4/1(q) -> Scope8/1, Display8/1
  PID Controller1/1 -> Model4/1(ua), comanda1/1
  Model4/2(h) -> Gain5/1, Display9/1, Scope9/1
  Gain5/1 -> Sum1/2
  Sum1/1 -> PID Controller1/1
  Gain6/1 -> Sum1/1
  h dorit1/1 -> Gain6/1
  Sum2/1 -> PID Controller2/1
  Model5/2(h) -> Gain7/1, Display11/1, Scope11/1
  h dorit2/1 -> Gain8/1
  Gain8/1 -> Sum2/1
  PID Controller2/1 -> Model5/1(ua), comanda2/1
  Model5/1(q) -> Scope10/1, Display10/1
  Gain7/1 -> Sum2/2
  Model6/1(q) -> Scope12/1, Display12/1
  PID Controller3/1 -> Model6/1(ua), comanda3/1
  Model6/2(h) -> Gain9/1, Display13/1, Scope13/1
  Gain9/1 -> Sum3/2
  Sum3/1 -> PID Controller3/1
  Gain10/1 -> Sum3/1
  h dorit3/1 -> Gain10/1
  Model6/3(qe) -> Scope14/1
  Model7/2(h) -> Gain12/1, Display15/1, Scope16/1
  PID Controller4/1 -> Model7/1(ua), comanda4/1
  h dorit4/1 -> Gain11/1
  Gain12/1 -> Sum4/2
  Sum4/1 -> PID Controller4/1
  Model7/3(perturbatia) -> Scope17/1
  Model7/1(q) -> Scope15/1, Display14/1
  Gain11/1 -> Sum4/1
  Model8/3(perturbatia) -> Gain15/1
  Gain13/1 -> Sum5/1
  Model8/1(q) -> Display16/1, Scope18/1
  Sum5/1 -> PID Controller5/1
  Gain14/1 -> Sum5/2
  h dorit5/1 -> Gain13/1
  Model8/2(h) -> Gain14/1, Display17/1, Scope19/1
  PID Controller5/1 -> Sum6/1
  Sum6/1 -> Model8/1(ua), comanda5/1
  Gain15/1 -> Sum6/2
  Curent/1(im) -> Motor/2(im)
  "Amplificator "/1(um) -> Randament/2(um), Curent/4(um), Motor/1(um)
  Randament/1(eta) -> Curent/2(eta)
  Filtru/1(q_f) -> Scope20/1, q/1, Rezervor/1(q_f), Curent/1(q_f), Randament/1(q_f)
  Motor/1(kn) -> Pompa/1(kn)
  Rezervor/1(h) -> h/1, Curent/3(h), Pompa/2(h)
  Pompa/1(q) -> Filtru/1(q)
  Step2/1 -> "Amplificator "/1(ua)
  Model process/2(h) -> Display19/1, Scope21/1
  Sum7/1 -> PID Controller6/1
  PID Controller6/1 -> Model process/1(ua)
  Model process/1(q) -> Sum7/2, Display18/1, Scope22/1
  Step3/1 -> Sum7/1
  Model process1/1(q) -> Sum8/2, Display20/1, Scope24/1
  Step4/1 -> Sum8/1
  Sum8/1 -> PID Controller7/1
  PID Controller7/1 -> Model process1/1(ua)
  Model process1/2(h) -> Display21/1, Scope23/1
  Model process2/2(h) -> Gain17/1, Display23/1, Scope25/1
  Gain16/1 -> Sum10/1
  PID Controller9/1 -> Sum9/1
  Step5/1 -> Gain16/1
  Gain17/1 -> Sum10/2
  Sum10/1 -> PID Controller9/1
  Model process2/1(q) -> Sum9/2, Display22/1, Scope26/1
  Sum9/1 -> PID Controller8/1
  Sum11/1 -> PID Controller11/1
  Step6/1 -> Gain18/1
  Gain19/1 -> Sum11/2
  PID Controller11/1 -> Sum12/1
  Gain18/1 -> Sum11/1
  Sum12/1 -> PID Controller10/1
  PID Controller10/1 -> Model9/1(ua)
  Model9/2(h) -> Gain19/1, Display25/1, Scope27/1
  Model9/1(q) -> Sum12/2, Display24/1, Scope28/1
  Sum14/1 -> PID Controller12/1
  Step7/1 -> Gain20/1
  Gain21/1 -> Sum13/2
  Gain20/1 -> Sum13/1
  Model10/1(q) -> Display26/1, Scope30/1, Sum14/3
  PID Controller12/1 -> Model10/1(ua)
  Model10/2(h) -> Gain21/1, Scope29/1, Display27/1
  Sum13/1 -> PID Controller13/1
  PID Controller13/1 -> Sum14/2
  Model10/3(perturbatia) -> Sum14/1
  Amplificator 1/1(um) -> To Workspace1/1, Scope34/1
  Ramp/1 -> To Workspace2/1, Scope35/1, Amplificator 1/1(ua)
  Constant/1 -> Rezervor1/1(q_f)
  Rezervor1/1(h) -> To Workspace3/1, Scope36/1
  PID Controller8/1 -> Model process2/1(ua)
  Model11/2(h) -> Gain1/1, Display29/1, Scope32/1
  h dorit6/1 -> Gain22/1
  Sum15/1 -> TCP/IP Send/1
  Model11/1(q) -> Scope31/1, Display28/1
  Gain22/1 -> Sum15/1
  Gain1/1 -> Sum15/2
  TCP/IP Receive/1 -> comanda6/1, IC/1
  IC/1 -> Model11/1(ua)

== system DatePersonalizate/Amplificator  ==
  ua : Inport
  Constant : Constant  Value=8.1
  Gain : Gain  Gain=2.2
  Gain1 : Gain  Gain=2.2
  Gain2 : Gain  Gain=5
  Saturation : Saturate  UpperLimit=22  LowerLimit=0
  Sum : Sum  Inputs=|++
  Sum1 : Sum  Inputs=|+-
  Switch : Switch  Criteria=u2 > Threshold  Threshold=8.1  SaturateOnIntegerOverflow=off  InputSameDT=off
  um : Outport
  wires:
  Gain2/1 -> Sum/2
  Gain1/1 -> Sum/1
  Sum1/1 -> Gain2/1
  Sum/1 -> Switch/1
  ua/1 -> Gain/1, Gain1/1, Sum1/1, Switch/2
  Constant/1 -> Sum1/2
  Gain/1 -> Switch/3
  Switch/1 -> Saturation/1
  Saturation/1 -> um/1

== system DatePersonalizate/Amplificator 1 ==
  ua : Inport
  Constant : Constant  Value=8.1
  Gain : Gain  Gain=2.2
  Gain1 : Gain  Gain=2.2
  Gain2 : Gain  Gain=5
  Saturation : Saturate  UpperLimit=22  LowerLimit=0
  Sum : Sum  Inputs=|++
  Sum1 : Sum  Inputs=|+-
  Switch : Switch  Criteria=u2 > Threshold  Threshold=8.1  SaturateOnIntegerOverflow=off  InputSameDT=off
  um : Outport
  wires:
  Gain2/1 -> Sum/2
  Gain1/1 -> Sum/1
  Sum1/1 -> Gain2/1
  Sum/1 -> Switch/1
  ua/1 -> Gain/1, Gain1/1, Sum1/1, Switch/2
  Constant/1 -> Sum1/2
  Gain/1 -> Switch/3
  Switch/1 -> Saturation/1
  Saturation/1 -> um/1

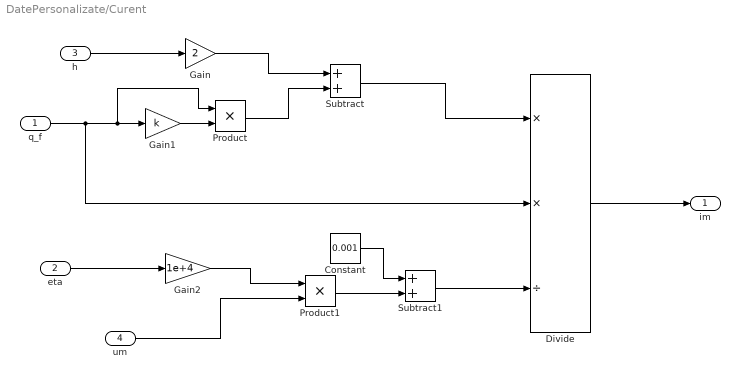
== system DatePersonalizate/Curent ==
  q_f : Inport
  eta : Inport  Port=2
  h : Inport  Port=3
  um : Inport  Port=4
  Constant : Constant  Value=0.001
  Divide : Product  Inputs=**/
  Gain : Gain  Gain=2
  Gain1 : Gain  Gain=k
  Gain2 : Gain  Gain=1e+4
  Product : Product
  Product1 : Product
  Subtract : Sum
  Subtract1 : Sum
  im : Outport
  wires:
  um/1 -> Product1/2
  h/1 -> Gain/1
  Product1/1 -> Subtract1/2
  eta/1 -> Gain2/1
  Gain/1 -> Subtract/1
  Constant/1 -> Subtract1/1
  Subtract/1 -> Divide/1
  Gain2/1 -> Product1/1
  Product/1 -> Subtract/2
  Subtract1/1 -> Divide/3
  q_f/1 -> Product/1, Gain1/1, Divide/2
  Divide/1 -> im/1
  Gain1/1 -> Product/2

== system DatePersonalizate/Filtru ==
  q : Inport
  Integrator1 : Integrator  InitialCondition=30.22
  Sum1 : Sum  Inputs=|+-
  q_f : Outport
  wires:
  Sum1/1 -> Integrator1/1
  q/1 -> Sum1/1
  Integrator1/1 -> q_f/1, Sum1/2

== system DatePersonalizate/Model process ==
  ua : Inport
  "Amplificator " : Subsystem
  Curent : Subsystem
  Filtru : Subsystem
  Motor : Subsystem
  Pompa : Subsystem
  Randament : Subsystem
  Rezervor : Subsystem
  q : Outport
  h : Outport  Port=2
  wires:
  ua/1 -> "Amplificator "/1(ua)
  Motor/1(kn) -> Pompa/1(kn)
  "Amplificator "/1(um) -> Curent/4(um), Randament/2(um), Motor/1(um)
  Rezervor/1(h) -> h/1, Curent/3(h), Pompa/2(h)
  Curent/1(im) -> Motor/2(im)
  Filtru/1(q_f) -> q/1, Rezervor/1(q_f), Curent/1(q_f), Randament/1(q_f)
  Randament/1(eta) -> Curent/2(eta)
  Pompa/1(q) -> Filtru/1(q)

== system DatePersonalizate/Model process1 ==
  ua : Inport
  "Amplificator " : Subsystem
  Curent : Subsystem
  Filtru : Subsystem
  Motor : Subsystem
  Pompa : Subsystem
  Randament : Subsystem
  Rezervor : Subsystem
  q : Outport
  h : Outport  Port=2
  wires:
  ua/1 -> "Amplificator "/1(ua)
  Motor/1(kn) -> Pompa/1(kn)
  "Amplificator "/1(um) -> Curent/4(um), Randament/2(um), Motor/1(um)
  Rezervor/1(h) -> h/1, Curent/3(h), Pompa/2(h)
  Curent/1(im) -> Motor/2(im)
  Filtru/1(q_f) -> q/1, Rezervor/1(q_f), Curent/1(q_f), Randament/1(q_f)
  Randament/1(eta) -> Curent/2(eta)
  Pompa/1(q) -> Filtru/1(q)

== system DatePersonalizate/Model process2 ==
  ua : Inport
  "Amplificator " : Subsystem
  Curent : Subsystem
  Filtru : Subsystem
  Motor : Subsystem
  Pompa : Subsystem
  Randament : Subsystem
  Rezervor : Subsystem
  q : Outport
  h : Outport  Port=2
  wires:
  ua/1 -> "Amplificator "/1(ua)
  Motor/1(kn) -> Pompa/1(kn)
  "Amplificator "/1(um) -> Curent/4(um), Randament/2(um), Motor/1(um)
  Rezervor/1(h) -> h/1, Curent/3(h), Pompa/2(h)
  Curent/1(im) -> Motor/2(im)
  Filtru/1(q_f) -> q/1, Rezervor/1(q_f), Curent/1(q_f), Randament/1(q_f)
  Randament/1(eta) -> Curent/2(eta)
  Pompa/1(q) -> Filtru/1(q)

== system DatePersonalizate/Model1 ==
  ua : Inport
  "Amplificator " : Subsystem
  Curent : Subsystem
  Filtru : Subsystem
  Motor : Subsystem
  Pompa : Subsystem
  Randament : Subsystem
  Rezervor : Subsystem
  q : Outport
  h : Outport  Port=2
  wires:
  ua/1 -> "Amplificator "/1(ua)
  Motor/1(kn) -> Pompa/1(kn)
  "Amplificator "/1(um) -> Curent/4(um), Randament/2(um), Motor/1(um)
  Rezervor/1(h) -> h/1, Curent/3(h), Pompa/2(h)
  Curent/1(im) -> Motor/2(im)
  Filtru/1(q_f) -> q/1, Rezervor/1(q_f), Curent/1(q_f), Randament/1(q_f)
  Randament/1(eta) -> Curent/2(eta)
  Pompa/1(qi) -> Filtru/1(qi)

== system DatePersonalizate/Model10 ==
  ua : Inport
  "Amplificator " : Subsystem
  Curent : Subsystem
  Filtru : Subsystem
  Motor : Subsystem
  Pompa : Subsystem
  Randament : Subsystem
  "Rezervor " : Subsystem
  Step : Step  Time=250  After=0.2*k  SampleTime=0
  q : Outport
  h : Outport  Port=2
  perturbatia : Outport  Port=3
  wires:
  ua/1 -> "Amplificator "/1(ua)
  Motor/1(kn) -> Pompa/1(kn)
  "Amplificator "/1(um) -> Curent/4(um), Randament/2(um), Motor/1(um)
  "Rezervor "/1(h) -> Pompa/2(h), Curent/3(h), h/1
  Curent/1(im) -> Motor/2(im)
  Filtru/1(q_f) -> q/1, "Rezervor "/1(q), Curent/1(q_f), Randament/1(q_f)
  Randament/1(eta) -> Curent/2(eta)
  Pompa/1(q) -> Filtru/1(q)
  Step/1 -> Pompa/3(perturbatia k)
  "Rezervor "/2(perturbatia) -> perturbatia/1

== system DatePersonalizate/Model11 ==
  ua : Inport
  "Amplificator " : Subsystem
  Curent : Subsystem
  Filtru : Subsystem
  Motor : Subsystem
  Pompa : Subsystem
  Randament : Subsystem
  Rezervor : Subsystem
  q : Outport
  h : Outport  Port=2
  wires:
  ua/1 -> "Amplificator "/1(ua)
  Motor/1(kn) -> Pompa/1(kn)
  "Amplificator "/1(um) -> Curent/4(um), Randament/2(um), Motor/1(um)
  Rezervor/1(h) -> h/1, Curent/3(h), Pompa/2(h)
  Curent/1(im) -> Motor/2(im)
  Filtru/1(q_f) -> q/1, Rezervor/1(q_f), Curent/1(q_f), Randament/1(q_f)
  Randament/1(eta) -> Curent/2(eta)
  Pompa/1(q) -> Filtru/1(q)

== system DatePersonalizate/Model2 ==
  ua : Inport
  "Amplificator " : Subsystem
  Curent : Subsystem
  Filtru : Subsystem
  Motor : Subsystem
  Pompa : Subsystem
  Randament : Subsystem
  Rezervor : Subsystem
  q : Outport
  h : Outport  Port=2
  wires:
  ua/1 -> "Amplificator "/1(ua)
  Motor/1(kn) -> Pompa/1(kn)
  "Amplificator "/1(um) -> Curent/4(um), Randament/2(um), Motor/1(um)
  Rezervor/1(h) -> h/1, Curent/3(h), Pompa/2(h)
  Curent/1(im) -> Motor/2(im)
  Filtru/1(q_f) -> q/1, Rezervor/1(q_f), Curent/1(q_f), Randament/1(q_f)
  Randament/1(eta) -> Curent/2(eta)
  Pompa/1(q) -> Filtru/1(q)

== system DatePersonalizate/Model3 ==
  ua : Inport
  "Amplificator " : Subsystem
  Curent : Subsystem
  Filtru : Subsystem
  Motor : Subsystem
  Pompa : Subsystem
  Randament : Subsystem
  Rezervor : Subsystem
  q : Outport
  h : Outport  Port=2
  wires:
  ua/1 -> "Amplificator "/1(ua)
  Motor/1(kn) -> Pompa/1(kn)
  "Amplificator "/1(um) -> Curent/4(um), Randament/2(um), Motor/1(um)
  Rezervor/1(h) -> h/1, Curent/3(h), Pompa/2(h)
  Curent/1(im) -> Motor/2(im)
  Filtru/1(q_f) -> q/1, Rezervor/1(q_f), Curent/1(q_f), Randament/1(q_f)
  Randament/1(eta) -> Curent/2(eta)
  Pompa/1(q) -> Filtru/1(q)

== system DatePersonalizate/Model4 ==
  ua : Inport
  "Amplificator " : Subsystem
  Curent : Subsystem
  Filtru : Subsystem
  Motor : Subsystem
  Pompa : Subsystem
  Randament : Subsystem
  Rezervor : Subsystem
  q : Outport
  h : Outport  Port=2
  wires:
  ua/1 -> "Amplificator "/1(ua)
  Motor/1(kn) -> Pompa/1(kn)
  "Amplificator "/1(um) -> Curent/4(um), Randament/2(um), Motor/1(um)
  Rezervor/1(h) -> h/1, Pompa/2(h), Curent/3(h)
  Curent/1(im) -> Motor/2(im)
  Filtru/1(q_f) -> q/1, Rezervor/1(q_f), Curent/1(q_f), Randament/1(q_f)
  Randament/1(eta) -> Curent/2(eta)
  Pompa/1(q) -> Filtru/1(q)

== system DatePersonalizate/Model5 ==
  ua : Inport
  "Amplificator " : Subsystem
  Curent : Subsystem
  Filtru : Subsystem
  Motor : Subsystem
  Pompa : Subsystem
  Randament : Subsystem
  Rezervor : Subsystem
  Step : Step  Time=250  After=0.2*k  SampleTime=0
  q : Outport
  h : Outport  Port=2
  wires:
  ua/1 -> "Amplificator "/1(ua)
  Motor/1(kn) -> Pompa/1(kn)
  "Amplificator "/1(um) -> Curent/4(um), Randament/2(um), Motor/1(um)
  Rezervor/1(h) -> h/1, Pompa/2(h), Curent/3(h)
  Curent/1(im) -> Motor/2(im)
  Filtru/1(q_f) -> q/1, Rezervor/1(q_f), Curent/1(q_f), Randament/1(q_f)
  Randament/1(eta) -> Curent/2(eta)
  Pompa/1(q) -> Filtru/1(q)
  Step/1 -> Pompa/3(perturbatia k)

== system DatePersonalizate/Model6 ==
  ua : Inport
  "Amplificator " : Subsystem
  Curent : Subsystem
  Filtru : Subsystem
  Motor : Subsystem
  Pompa : Subsystem
  Randament : Subsystem
  "Rezervor " : Subsystem
  q : Outport
  h : Outport  Port=2
  qe : Outport  Port=3
  wires:
  ua/1 -> "Amplificator "/1(ua)
  Motor/1(kn) -> Pompa/1(kn)
  "Amplificator "/1(um) -> Curent/4(um), Randament/2(um), Motor/1(um)
  "Rezervor "/1(h) -> h/1, Curent/3(h), Pompa/2(h)
  Curent/1(im) -> Motor/2(im)
  Filtru/1(q_f) -> q/1, "Rezervor "/1(q), Curent/1(q_f), Randament/1(q_f)
  Randament/1(eta) -> Curent/2(eta)
  Pompa/1(q) -> Filtru/1(q)
  "Rezervor "/2(qe) -> qe/1

== system DatePersonalizate/Model7 ==
  ua : Inport
  "Amplificator " : Subsystem
  Curent : Subsystem
  Filtru : Subsystem
  Motor : Subsystem
  Pompa : Subsystem
  Randament : Subsystem
  "Rezervor " : Subsystem
  q : Outport
  h : Outport  Port=2
  perturbatia : Outport  Port=3
  wires:
  ua/1 -> "Amplificator "/1(ua)
  Motor/1(kn) -> Pompa/1(kn)
  "Amplificator "/1(um) -> Curent/4(um), Randament/2(um), Motor/1(um)
  "Rezervor "/1(h) -> h/1, Curent/3(h), Pompa/2(h)
  Curent/1(im) -> Motor/2(im)
  Filtru/1(q_f) -> "Rezervor "/1(q), q/1, Curent/1(q_f), Randament/1(q_f)
  Randament/1(eta) -> Curent/2(eta)
  Pompa/1(q) -> Filtru/1(q)
  "Rezervor "/2(perturbatia) -> perturbatia/1

== system DatePersonalizate/Model8 ==
  ua : Inport
  "Amplificator " : Subsystem
  Curent : Subsystem
  Filtru : Subsystem
  Motor : Subsystem
  Pompa : Subsystem
  Randament : Subsystem
  "Rezervor " : Subsystem
  q : Outport
  h : Outport  Port=2
  perturbatia : Outport  Port=3
  wires:
  ua/1 -> "Amplificator "/1(ua)
  Motor/1(kn) -> Pompa/1(kn)
  "Amplificator "/1(um) -> Curent/4(um), Randament/2(um), Motor/1(um)
  "Rezervor "/1(h) -> h/1, Curent/3(h), Pompa/2(h)
  Curent/1(im) -> Motor/2(im)
  Filtru/1(q_f) -> "Rezervor "/1(q), q/1, Curent/1(q_f), Randament/1(q_f)
  Randament/1(eta) -> Curent/2(eta)
  Pompa/1(q) -> Filtru/1(q)
  "Rezervor "/2(perturbatia) -> perturbatia/1

== system DatePersonalizate/Model9 ==
  ua : Inport
  "Amplificator " : Subsystem
  Curent : Subsystem
  Filtru : Subsystem
  Motor : Subsystem
  Pompa : Subsystem
  Randament : Subsystem
  Rezervor : Subsystem
  Step : Step  Time=250  After=0.2*k  SampleTime=0
  q : Outport
  h : Outport  Port=2
  wires:
  ua/1 -> "Amplificator "/1(ua)
  Motor/1(kn) -> Pompa/1(kn)
  "Amplificator "/1(um) -> Curent/4(um), Randament/2(um), Motor/1(um)
  Rezervor/1(h) -> h/1, Pompa/2(h), Curent/3(h)
  Curent/1(im) -> Motor/2(im)
  Filtru/1(q_f) -> q/1, Rezervor/1(q_f), Curent/1(q_f), Randament/1(q_f)
  Randament/1(eta) -> Curent/2(eta)
  Pompa/1(q) -> Filtru/1(q)
  Step/1 -> Pompa/3(perturbatia k)

== system DatePersonalizate/Motor ==
  um : Inport
  im : Inport  Port=2
  Add : Sum  Inputs=+-
  Gain : Gain  Gain=3
  kn : Outport
  wires:
  Gain/1 -> Add/2
  im/1 -> Gain/1
  um/1 -> Add/1
  Add/1 -> kn/1

== system DatePersonalizate/Pompa ==
  kn : Inport
  h : Inport  Port=2
  Gain : Gain  Gain=1/k13
  Gain1 : Gain  Gain=k2
  Gain2 : Gain  Gain=k11
  Gain3 : Gain  Gain=k12
  Product : Product
  Sqrt : Sqrt
  Subtract : Sum
  Subtract1 : Sum  Inputs=+-
  q : Outport
  wires:
  Subtract/1 -> Gain/1
  Sqrt/1 -> Subtract/2
  kn/1 -> Product/2, Product/1, Gain1/1
  Gain3/1 -> Subtract1/2
  Subtract1/1 -> Sqrt/1
  Gain1/1 -> Subtract/1
  h/1 -> Gain3/1
  Product/1 -> Gain2/1
  Gain2/1 -> Subtract1/1
  Gain/1 -> q/1

== system DatePersonalizate/Randament ==
  q_f : Inport
  um : Inport  Port=2
  Gain : Gain  Gain=keta
  Product : Product
  eta : Outport
  wires:
  Gain/1 -> Product/2
  um/1 -> Gain/1
  q_f/1 -> Product/1
  Product/1 -> eta/1

== system DatePersonalizate/Rezervor ==
  q_f : Inport
  Fcn : Fcn  Expr=sqrt(u)*C
  Gain : Gain  Gain=1/S
  Integrator : Integrator  InitialCondition=16.53
  Sum : Sum  Inputs=|+-
  h : Outport
  wires:
  Gain/1 -> Integrator/1
  q_f/1 -> Sum/1
  Integrator/1 -> h/1, Fcn/1
  Sum/1 -> Gain/1
  Fcn/1 -> Sum/2

== system DatePersonalizate/Rezervor1 ==
  q_f : Inport
  Fcn : Fcn  Expr=sqrt(u)*9
  Gain : Gain  Gain=1/S
  Integrator : Integrator  InitialCondition=17
  Scope : Scope
  Sum : Sum  Inputs=|+-
  To Workspace : ToWorkspace  VariableName=debit_iesire  SampleTime=-1
  h : Outport
  wires:
  Gain/1 -> Integrator/1
  q_f/1 -> Sum/1
  Integrator/1 -> h/1, Fcn/1
  Sum/1 -> Gain/1
  Fcn/1 -> To Workspace/1, Scope/1, Sum/2
